simulink model "Plant"  (R2025a)
settings: Solver=ode4  StartTime=0.0  StopTime=10  FixedStep=2e-4  RelTol=1e-3
model workspace (MAT data in the model file):
  phTyreNomPres = 262000
  plantVx0 = 68.8718280662
undefined symbols (not defined in the file): pt, sus, tyreParamVec, vp
libraries: AeroActuators x2, vehdynlibeom x1
(part 1 of 2)
Description:
  | ARFWr RT plant (T2.2 skeleton). 1 kHz, ode4, model-reference target for ARFWr_Sim.
  | 
  | FRAME CONVENTION -- READ FIRST.
  | The rigid body is the VDB "Vehicle Body 6DOF" block, which wraps the Aerospace
  | 6DOF (Euler Angles) block and therefore uses SAE J670 body axes: x FORWARD,
  | y RIGHT, z DOWN. This was MEASURED on the live R2025a block during T2.2, not
  | assumed: FSusp(3,:) = -[Ff Ff Fr Fr] holds the body in exact static equilibrium
  | (all six DOF stay at zero), while +z of the same magnitude doubles the
  | gravitational fall. FSusp/MSusp are 3-by-4, columns ordered [FL FR RL RR]
  | (measured: an extra UP force on column 1 rolls the body left-side-up).
  | 
  | Everything else in this repo -- Scripts/vehModel.m, the ARFWr reactive law,
  | simulink/ecu/tvAllocStep.m, the curv2cart racing line -- is ISO 8855:
  | x FORWARD, y LEFT, z UP, yaw rate r > 0 = LEFT turn.
  | 
  | This model therefore works INTERNALLY in the SAE frame and MIRRORS at the bus
  | boundary (Vehicle State Bus subsystem):  y, vy, ay, psi, r, z, roll all negate;
  | pitch does not (the mirror is about the x-z plane). Corner LABELS fl/fr/rl/rr
  | are physical and never flip.
  | 
  | PLACEHOLDERS in this model (see the model workspace, all prefixed ph*):
  |   phTyreNomPres        tyre block nominal pressure (inert: driven AT NOMPRES)
  | T3.2 replaced the tyre placeholder with the Zenvo MF5.2 law; T3.4 replaced the aero placeholder with the live ride-height map, so the constant-coefficient phAeroClF/phAeroClR and the phIxx/phIyy inertia placeholders are deleted -- the inertia tensor is now the supplier one (inrt.Iveh).
settings Model: DataDictionary=ARFWr_RT.sldd  Creator=ASUS  LastModifiedBy=ASUS
settings DataIOCC: SignalLoggingName=plantLog
settings DebuggingCC: AlgebraicLoopMsg=error  UnconnectedInputMsg=error  UnconnectedOutputMsg=error  UnconnectedLineMsg=error

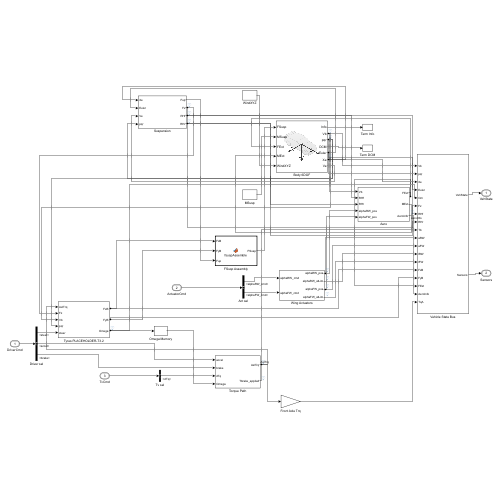
[thumbnail: Simulink's stored preview of the top-level diagram]
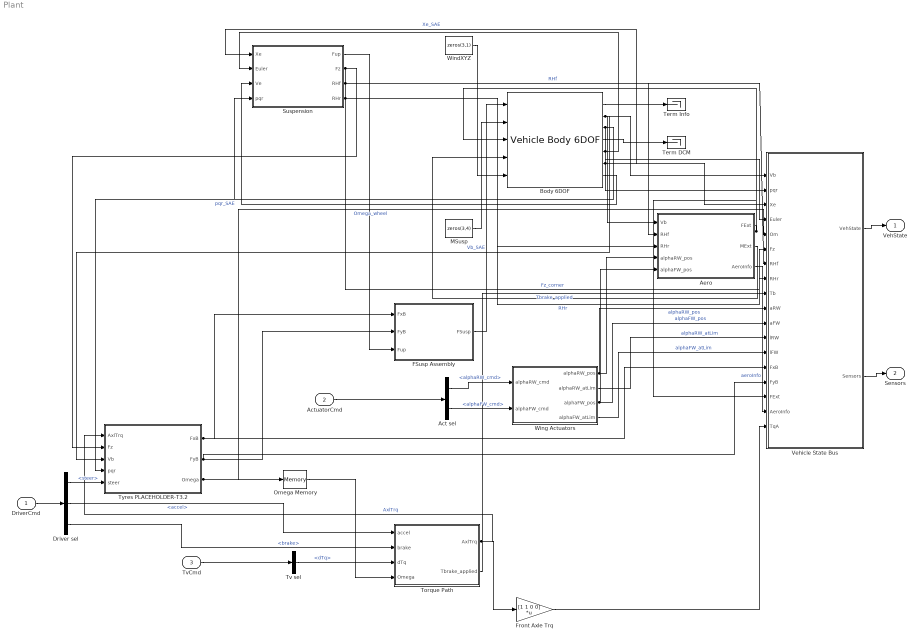
== system Plant ==
  DriverCmd : Inport  Description=Driver / scenario demand. ISO 8855 steer (+ = LEFT road-wheel angle, rad), accel and brake in 0..1.  OutDataTypeStr=Bus: DriverCmdBus
  ActuatorCmd : Inport  Description=Wing angle demands out of AeroECU. The two wing ACTUATORS live here in the plant (design decision 7: they are the HIL seam, replaced by hardware later), so the ECU commands and the plant reports positions.  Port=2  OutDataTypeStr=Bus: ActuatorCmdBus
  TvCmd : Inport  Description=Torque-vectoring differential torque (TvCmdBus.dTq), driven by the AeroECU allocator in the closed-loop harness. The Torque Path applies it as a front-axle left/right split: AxlTrq_FR - AxlTrq_FL = dTq.  Port=3  OutDataTypeStr=Bus: TvCmdBus
  Act sel : BusSelector  OutputSignals=alphaRW_cmd,alphaFW_cmd
  Aero : Subsystem  Description=|
      | LIVE ride-height aerodynamics (T3.4). Replaced the T2.2 constant-coefficient placeholder; the four signals that used to be terminated here (RHf, RHr, alphaRW_pos, alphaFW_pos) are now CONSUMED, so the wings finally do something.
      | 
      | WHAT IT COMPUTES, per step (formulas and derivation: simulink/aero/aeroLiveEval.m):
      |   ClF = interp2(base map)(RHf,RHr) + blend_RW(alphaRW).dClF + blend_FW(alphaFW).dClFadd
      |   ClR = interp2(base map)(RHf,RHr) + blend_RW(alphaRW).dClR + blend_FW(alphaFW).dClRadd
      |   Cd  = vp.Cd0 + (dCdA_RW(alphaRW) + dCdA_FW(alphaFW))/vp.A
      | The base map is the MID (0 deg both wings) ride-height grid, indexed at the INSTANTANEOUS ride height the Suspension subsystem publishes -- not at a quasi-statically collapsed one. That is the whole reason a 6-DOF plant is worth building: the offline solver bakes ride height out of the model (one aeroCollapse fixed point per wing node, fitted to a speed-only curve), and cannot see a transient attitude.
      | 
      | FORCE APPLICATION (SAE body axes here: x fwd, y RIGHT, z DOWN).
      | FExt acts at the CG (measured on the VDB block in T2.2: an FExt(1) step produces exactly zero pitch), so both the front/rear lift split AND the drag height split have to be re-expressed as explicit MExt pitch moments:
      |   lift  DFf at x = +vp.l_f, DFr at x = -vp.l_r   ->  M_y = -l_f*DFf + l_r*DFr
      |   drag  body part vp.Cd0 at vp.hcg  ->  no moment (it acts at the CG height)
      |         wing increment (Cd - Cd0) at vp.hw  ->  M_y = +(vp.hw - vp.hcg)*Fdrag_rw
      | This is the vp.hw term build_plant.m's placeholder description said T3.4 would add, and it is the same f_drag0/f_dragRW height split Scripts/vehModel.m:603-604 defines.
      | 
      | KNOWN LIMITATION, read before believing a deployed-front-wing number. The offline model builds the FRONT-wing layer with liftMode = 'additive' (Functions/rwAeroMap2D.m), i.e. the FW lift deltas are added to a ride-height trajectory collapsed with the FW delta set to ZERO -- deliberately, because the FW-deployed CFD states fall outside aeroCollapse's convergence envelope. A live plant cannot open that loop: here the FW lift delta really does extend the front suspension, which raises the nose, which the base map answers with LESS front downforce. See docs / the T3.4 report for the measured size of that divergence.
  Body 6DOF : vehdynlibeom/Vehicle Body 6DOF  Description=|  extPos=on  extVel=on  extEuler=on  extRotRate=on  htchFMode=off  htchMMode=off  m=vp.m  a=vp.l_f  b=vp.l_r  d=0  h=vp.hcg  dh=1  hl=0  hh=0.1  Xe_o=[0,0,0]  xbdot_o=[plantVx0,0,0]  eul_o=[0,0,0]  p_o=[0,0,0]  Iveh=inrt.Iveh  w=[vp.t, vp.t]  z1m=0  z1R=[-.25,.125,.15]  z1I=[1.4,-.2,.1;-.2,1.4,.1;.1,.1,2.25].*0  z2m=0  z2R=[1.4,0,.8]  z2I=[1.4,-.2,.1;-.2,1.4,.1;.1,.1,2.25].*0  z3m=0  z3R=[.75,-.5,.4]  z3I=[5,-.1,-2;-2,9,.1;-.1,.1,6].*0  z4m=0  z4R=[.75,.5,.4]  z4I=[5,-.1,-2;-2,9,.1;-.1,.1,6].*0  z5m=0  z5R=[1.25,-.5,.4]  z5I=[5,-.1,-2;-2,9,.1;-.1,.1,6].*0  z6m=0  z6R=[1.25,-.5,.4]  z6I=[5,-.1,-2;-2,9,.1;-.1,.1,6].*0  z7m=0  z7R=[2,0,.25]  z7I=[1.4,-.2,.1;-.2,1.4,.1;.1,.1,2.25].*0  Af=vp.A  Cd=0  Cl=0  Cpm=0  beta_w=[0:0.001:0.01]  Cs=[0:0.01:0.1]  Cym=[0:0.001:0.01]  Pabs=101325  extTamb=off  Tair=273  g=vp.g  xdot_tol=.1  longOff=0  latOff=0  vertOff=0  wrapAng=on  aMode=2
      | VDB Vehicle Body 6DOF -- SAE J670 body axes (x fwd, y RIGHT, z DOWN), measured in T2.2. See the model description for the full convention note.
      | 
      | h = vp.hcg (not vp.hcg - vp.Rw) ON PURPOSE. The mask calls h the "vertical distance from centre of mass to axle plane", i.e. the height at which FSusp columns are applied. This model has no unsprung mass and no suspension block, so what is fed through FSusp rows 1-2 is the TYRE CONTACT-PATCH force, whose true application height is ground level = vp.hcg below the CG. Setting h = vp.hcg therefore gives the correct roll/pitch moment arm (verified: a pure -x force at the corners produces nose-down pitch; a +y force rolls the body left-side-down, i.e. outboard).
      | 
      | The block's OWN aero model is switched off (Cd = Cl = Cpm = 0) so the Aero subsystem is the single owner of aerodynamic force -- otherwise T3.4 would have to fight a second, single-point aero model that cannot split lift per axle. Af is still set to vp.A so a reader sees the right reference area.
      | 
      | Iveh = inrt.Iveh (T3.4), the SUPPLIER tensor diag([500 2500 2900]) kg.m^2 from Zenvo's vehicle-parameter workbook, sheet "Vehicle", "Vehicle Inertia" rows 32-34. The T2.2 phIxx/phIyy placeholders are gone: they were built on the premise that no supplier Ixx/Iyy existed, and it does -- see simulink/params/inertiaBorrowed.m, which also carries the radius-of-gyration cross-check (a calibrated solid box predicts the two to within +1.5 % and +4.0 %). vp.I_z (2900) is the Izz entry of that same row block, so all three now come from one source.
  Driver sel : BusSelector  OutputSignals=steer,accel,brake
  FSusp Assembly : MATLAB Function  Description=Builds the VDB Vehicle Body 6DOF FSusp input: a 3-by-4 matrix, rows = force along vehicle-fixed [x; y; z], columns = [FL FR RL RR] (both MEASURED on the live block, see the model description). Rows 1-2 are the tyre contact-patch forces in body axes; row 3 is -Fup, because the suspension pushes the body UP and +z is DOWN.  TreatAsAtomicUnit=on
  Front Axle Trq : Gain  Description=|  Gain=[1 1 0 0]  Multiplication=Matrix(K*u)
      | TqAxle for the TV allocator: the NOMINAL (pre-TV) total FRONT-axle wheel torque,
      | AxlTrq(FL) + AxlTrq(FR), in Nm, drive plus brake, signed.
      | 
      | WHY THE SUM IS THE PRE-TV QUANTITY, exactly and not approximately: Torque Path's
      | torqueStep forms AxlTrq(1) = TwF/2 - dTq/2 + Tbf and AxlTrq(2) = TwF/2 + dTq/2 + Tbf,
      | so the +/-dTq/2 shift CANCELS in the sum by construction and this signal equals
      | TwF + 2*Tbf for any dTq. That is precisely what simulink/ecu/tvAllocStep.m's headroom
      | clamp expects -- headroom = 2*(perSideCapNm - |TqAxle|/2) is the room each side has
      | left ABOVE its symmetric TqAxle/2 baseline -- so feeding the post-TV per-wheel torque
      | instead would double-count the shift the clamp is sizing.
      | 
      | It carries the BRAKE share too (Tbf), not just the drive share, because the per-wheel
      | motor torque a TV shift has to fit alongside is the whole signed wheel torque.
      | 
      | ALGEBRAIC LOOP: this closes dTq -> Torque Path -> here -> SensorBus -> ECU -> dTq. It
      | is broken OUTSIDE the Plant, by the one-sample Memory in ARFWr_Sim/ECU Sensor Latency
      | (the same block that already breaks the vx/r path), not by anything here.
  MSusp : Constant  Description=Suspension MOMENTS about each hard point. Zero: this skeleton applies pure forces at the contact patches, and the resulting body moments come from the hard-point lever arms the block already applies.  Value=zeros(3,4)
  Omega Memory : Memory  Description=|
      | ALGEBRAIC-LOOP BREAK. The VDB Combined Slip Wheel 2DOF block's Omega output has direct feedthrough from its AxlTrq input (through the block's own Wheel Module clutch), so feeding Omega back into the Torque Path's power cap closes an algebraic loop that Simulink refuses to solve (the clutch updates state while computing outputs).
      | 
      | Breaking it with a one-major-step Memory is both the standard fix and the physically honest one: the power cap min(Tmax*gear, Pmax/mean(Om)) is an inverter/ECU calculation that in hardware necessarily uses the PREVIOUS speed sample. At 1 ms the lag is negligible against wheel-speed dynamics, and the formula itself is unchanged from Scripts/vehModel.m:655 + Parameters/Powertrain.m:12. Initial condition 0 rad/s is the standstill state, where the cap is the torque branch (Tmax*gear) anyway -- the Om floor in torqueStep guards the division.
  Suspension : Subsystem  Description=|
      | Four independent corners: linear wheel-rate spring (vp.kwf/vp.kwr), borrowed damper (sus.cDamp_f/sus.cDamp_r) and borrowed anti-roll bar (sus.kArb_f/sus.kArb_r) -- see simulink/params/suspensionBorrowed.m for the OptimumG derivation and provenance tags.
      | 
      | MODELLING LIMITATION (skeleton): rigid tyres, no unsprung mass, no tyre vertical stiffness, flat ground, and no roll-centre/jacking geometry. Corner compression is purely the body attitude change at that corner, so load transfer here is the through-the-springs component only. The geometric (roll-centre) component is missing; vp.hRCf/vp.hRCr exist and a later task can add it. Also: the model starts in exact static equilibrium (the static corner load is carried explicitly), so compression = 0 IS the reference attitude and RHf/RHr start at vp.RHf0/vp.RHr0.
      | 
      | RIDE HEIGHT UNITS: vp.RHf0 = 85 and vp.RHr0 = 95 are MILLIMETRES (Parameters/vehParams.m; Functions/aeroCollapse.m:23-25 documents the map grid as mm). Compression is metres, hence the x1000. CLOSED IN T3.4: the Params constant now carries vp.RHfU/vp.RHrU (the v = 0 unloaded heights) instead of vp.RHf0/vp.RHr0 (the v = 10 m/s nominal heights), so zero compression means the same physical attitude here as in Functions/aeroCollapse.m.
  Term DCM : Terminator
  Term Info : Terminator
  Torque Path : Subsystem  Description=|
      | Simplified torque path, mirroring Scripts/vehModel.m:660-663 (the pt.ATD == 0 ladder) plus the front-axle TV shift of simulink/ecu/tvAllocStep.m.
      | SOURCES OF THE TWO SPLIT CONSTANTS (found by grep for T2.2 -- pt.ATD is NOT set by Parameters/Powertrain.m, it is set by Scripts/userOpts.m, so the plant reproduces the fixed AWD split, not an ATD ladder):
      |   vp.Tdist = 0.78  Parameters/vehParams.m:20 -- REAR torque fraction. Sized in Parameters/Powertrain.m:71-75 so the fixed split never demands more than the front axle's 300 kW (2 x 150 kW e-motors) out of the 1068 kW rear path.
      |   vp.brkB  = 0.65  Parameters/vehParams.m:19 -- FRONT brake-force fraction, Zenvo sheet "mechanical pressure bias front 0.65 nominally".
      | Both are read by NAME from the base workspace via the Params constant.
  Tv sel : BusSelector  OutputSignals=dTq
  Tyres PLACEHOLDER-T3.2 : Subsystem  Description=|
      | TYRES -- real Zenvo MF5.2, applied T3.2. (The block name still carries the PLACEHOLDER-T3.2 tag only because renaming a subsystem breaks every stored signal-logging path and every task brief that references it.)
      | 
      | The four VDB "Combined Slip Wheel 2DOF" blocks are GONE, replaced by tyreStep, a direct implementation of Functions/tyreMFnum.m, plus an explicit wheel-spin integrator. See tyreStep's own description for the measured gate-1 evidence that forced this, and TyreParams for how the confidential coefficients reach the model without being stored in it.
      | 
      | --- superseded notes from the placeholder era, kept for provenance ---
      | *** PLACEHOLDER-T3.2 *** The two VDB "Combined Slip Wheel 2DOF" blocks inside carry their BUILT-IN DEFAULT Magic Formula 6.2 coefficient set (the block's "Mid-size passenger car 235/45R18"), NOT the Zenvo MF5.2 data. Peak mu is therefore about 0.81 and the car is far less grippy than the real vehicle. T3.2 replaces exactly this: mf52ToVDB(vp.tyre_f) / mf52ToVDB(vp.tyre_r) set_param'd onto the two blocks -- one block per axle is deliberate, because that is the granularity of the supplier data (vp.tyre_f / vp.tyre_r). THE SWAP IS ONE SUBSYSTEM: nothing outside this boundary changes.
      | 
      | CONFIDENTIALITY: no tyre coefficient value is stored in this .slx. T3.2 must apply them by set_param from vp.tyre_f/vp.tyre_r at load time, or the .slx would carry supplier data in its dialogs (project confidentiality rule).
      | 
      | STRUCTURAL settings applied here (vehicle geometry / wiring choices, NOT tyre data, and identical to what simulink/validation/validateTyreBlocks.m sets for gate 1): vertType = None (normal load comes in through Fext, so the suspension owns the vertical chain), BrakeType = None (brake torque is carried signed inside AxlTrq, matching vehModel.m's T_fl..T_rr), turnslip = off, and a rigid effective rolling radius equal to vp.Rw (UNLOADED_RADIUS = vp.Rw, Q_RE0 = 1, BREFF = DREFF = FREFF = 0). IYY is set to vp.Jw so wheel spin-up matches the MLTP model. plySteer is also OFF: the default tyre's ply-steer/conicity shift terms (PHY1, PVY1, ...) are identical on both sides of the car, so they push a nominally symmetric straight-line run sideways -- measured in T2.2, the untouched default reached |vy| = 11.8 m/s and |r| = 3.2 rad/s on a zero-steer full-throttle run. mf52ToVDB.m sets every shift term to exactly zero anyway, so turning ply steer off makes the placeholder STRUCTURALLY match what T3.2 installs.
      | 
      | LIBRARY PATH NOTE for T3.2: the loadable path is 'vehdynlibtire/Combined Slip Wheel 2DOF'. The path currently hardcoded in validateTyreBlocks.m:299, 'vdynblks/Wheels and Tires/Combined Slip Wheel 2DOF', does NOT load in R2025a (there is no loadable block diagram named vdynblks) -- that is its own VERIFY #1 and must be fixed before gate 1 runs.
      | 
      | T3.2 WIRING FIX (2026-09-02) -- MEASURED ROOT CAUSE.
      | Setting BrakeType = 'None' does TWO things to this block's input port list: it
      | removes BrkPrs (10 ports -> 9) AND it SWAPS the relative order of Gnd and Fext.
      | Measured on the live R2025a block:
      |   defaults           (10): BrkPrs AxlTrq Vx Vy Camber YawRate Prs Gnd Fext ScaleFctrs
      |   BrakeType = None    (9): AxlTrq Vx Vy Camber YawRate Prs Fext Gnd ScaleFctrs
      | build_plant.m accounted for the dropped BrkPrs but not the swap, so it wired the
      | Gnd constant (0) into port 7 = Fext and the suspension normal load DFzc into
      | port 8 = Gnd. With vertType = None the Gnd input is inert, so every tyre ran at
      | Fz = 0 (T2.3 measured tyre Fz output exactly 0.0 while VehStateBus.Fz_rl read
      | 4479-5085 N), produced ~30-100 N instead of thousands, and the wheels spun up
      | until the My Relaxation integrator went non-finite (t = 0.1825 s at 25%% throttle
      | from rest -- re-measured on the committed file by T3.2).
      | Ports 7/8 are now DFzc -> Fext, Gnd constant -> Gnd, and each block's own Fz
      | output is NAMED and LOGGED (Fz_tyre_FL..RR) so this class of fault is visible.
      | NEVER wire this block by port NUMBER against the documented order: resolve the
      | index from the live port names (find_system for its internal Inport blocks).
  Vehicle State Bus : Subsystem  Description=|
      | Assembles VehStateBus and SensorBus, and applies the SAE -> ISO 8855 mirror documented in the model description. This subsystem is the ONLY place the sign flip happens; nothing downstream (AeroECU, DriverPath, the reactive law, the TV allocator) ever sees SAE-framed signals.
      | 
      | SensorBus contract, checked against Functions/rwVelocityTarget.m's brakeSwitch: Tbrake is passed SIGNED (<= 0 while braking) -- brakeSwitch applies tbSign = -1 itself and deliberately avoids abs() -- and TbMax is the POSITIVE magnitude cap vp.Tbrake_max = 7000 Nm. TbMax > 0 ALWAYS: the law's onset width is w1frac*TbMax, so a negative or zero TbMax would invert or divide-by-zero the brake trigger.
  WindXYZ : Constant  Description=Wind velocity [m/s]. Zero: still air.  Value=zeros(3,1)
  Wing Actuators : Subsystem  Description=Both wing actuators: first-order lag (act.tau) -> rate limit (act.rateLim, +-25 deg/s Zenvo directive) -> travel clamp. Library instances of AeroActuators/ActuatorWing (T1.4). Positions are LOGGED and published on VehStateBus; T2.2 does NOT feed them to the aero -- the Aero subsystem receives them and terminates them, which is the seam T3.4 opens.
  VehState : Outport  Description=Full plant state, ISO 8855. See the sldd bus description.  OutDataTypeStr=Bus: VehStateBus
  Sensors : Outport  Description=The four signals AeroECU consumes, ISO 8855, Tbrake SIGNED.  Port=2  OutDataTypeStr=Bus: SensorBus
  wires:
  Omega Memory/1 -> Torque Path/4(Omega)
  DriverCmd/1 -> Driver sel/1
  TvCmd/1 -> Tv sel/1
  Driver sel/1 -> Tyres PLACEHOLDER-T3.2/5(steer)  "<steer>"
  Driver sel/2 -> Torque Path/1(accel)  "<accel>"
  Suspension/4(RHr) -> Aero/3(RHr), Vehicle State Bus/8(RHr)  "RHr"
  Tyres PLACEHOLDER-T3.2/2(FyB) -> FSusp Assembly/2(FyB), Vehicle State Bus/15(FyB)
  Wing Actuators/1(alphaRW_pos) -> Vehicle State Bus/10(aRW), Aero/4(alphaRW_pos)  "alphaRW_pos"
  Body 6DOF/7 -> Suspension/3(Ve)
  Tyres PLACEHOLDER-T3.2/1(FxB) -> Vehicle State Bus/14(FxB), FSusp Assembly/1(FxB)
  Body 6DOF/3 -> Suspension/4(pqr), Vehicle State Bus/2(pqr), Tyres PLACEHOLDER-T3.2/4(pqr)  "pqr_SAE"
  Driver sel/3 -> Torque Path/2(brake)  "<brake>"
  Tyres PLACEHOLDER-T3.2/3(Omega) -> Vehicle State Bus/5(Om), Omega Memory/1  "Omega_wheel"
  Suspension/1(Fup) -> FSusp Assembly/3(Fup)
  Suspension/2(Fz) -> Tyres PLACEHOLDER-T3.2/2(Fz), Vehicle State Bus/6(Fz)  "Fz_corner"
  Suspension/3(RHf) -> Aero/2(RHf), Vehicle State Bus/7(RHf)  "RHf"
  ActuatorCmd/1 -> Act sel/1
  Torque Path/1(AxlTrq) -> Tyres PLACEHOLDER-T3.2/1(AxlTrq), Front Axle Trq/1  "AxlTrq"
  Tv sel/1 -> Torque Path/3(dTq)  "<dTq>"
  WindXYZ/1 -> Body 6DOF/5
  MSusp/1 -> Body 6DOF/2
  FSusp Assembly/1(FSusp) -> Body 6DOF/1
  Vehicle State Bus/1(VehState) -> VehState/1
  Act sel/1 -> Wing Actuators/1(alphaRW_cmd)  "<alphaRW_cmd>"
  Act sel/2 -> Wing Actuators/2(alphaFW_cmd)  "<alphaFW_cmd>"
  Torque Path/2(Tbrake_applied) -> Vehicle State Bus/9(Tb)  "Tbrake_applied"
  Aero/2(MExt) -> Body 6DOF/4
  Body 6DOF/1 -> Term Info/1
  Body 6DOF/2 -> Tyres PLACEHOLDER-T3.2/3(Vb), Aero/1(Vb), Vehicle State Bus/1(Vb)  "Vb_SAE"
  Body 6DOF/4 -> Term DCM/1
  Body 6DOF/5 -> Suspension/2(Euler), Vehicle State Bus/4(Euler)
  Body 6DOF/6 -> Suspension/1(Xe), Vehicle State Bus/3(Xe)  "Xe_SAE"
  Wing Actuators/2(alphaRW_atLim) -> Vehicle State Bus/12(lRW)  "alphaRW_atLim"
  Wing Actuators/3(alphaFW_pos) -> Vehicle State Bus/11(aFW), Aero/5(alphaFW_pos)  "alphaFW_pos"
  Wing Actuators/4(alphaFW_atLim) -> Vehicle State Bus/13(lFW)  "alphaFW_atLim"
  Aero/1(FExt) -> Body 6DOF/3, Vehicle State Bus/16(FExt)
  Vehicle State Bus/2(Sensors) -> Sensors/1
  Aero/3(AeroInfo) -> Vehicle State Bus/17(AeroInfo)  "aeroInfo"
  Front Axle Trq/1 -> Vehicle State Bus/18(TqA)

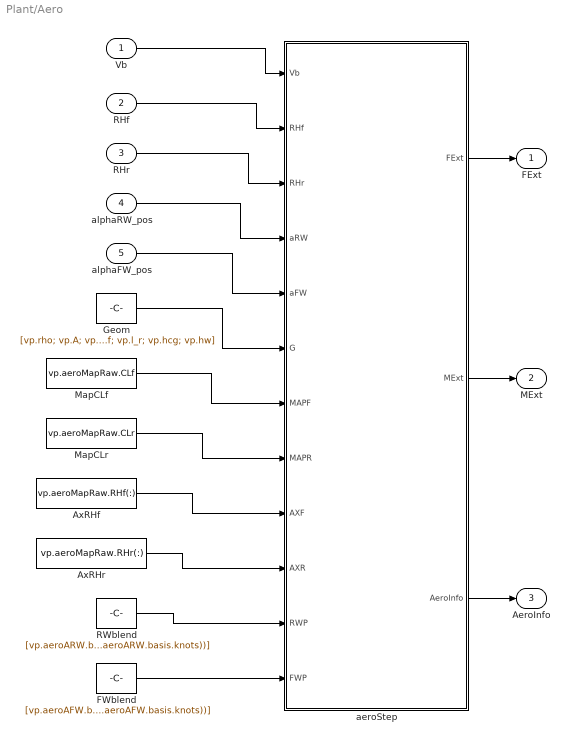
== system Plant/Aero ==
  Vb : Inport
  RHf : Inport  Port=2
  RHr : Inport  Port=3
  alphaRW_pos : Inport  Port=4
  alphaFW_pos : Inport  Port=5
  AxRHf : Constant  Description=Front ride-height axis of the raw map [mm], ascending. Grid edges are where aeroStep clamps.  Value=vp.aeroMapRaw.RHf(:)
  AxRHr : Constant  Description=Rear ride-height axis of the raw map [mm], ascending.  Value=vp.aeroMapRaw.RHr(:)
  FWblend : Constant  Description=|  Value=[vp.aeroAFW.basis.knots(:).'; repmat(vp.aeroAFW.basis.wb,1,numel(vp.aeroAFW.basis.knots)); vp.aeroAFW.dClFadd(:).'; vp.aeroAFW.dClRadd(:).'; vp.aeroAFW.dCdA(:).'; reshape(permute(vp.aeroAFW.basis.C,[2 1 3]),[],numel(vp.aeroAFW.basis.knots))]
      | Cardinal-basis blend parameters for the FRONT wing, packed as a matrix with one COLUMN per map node. Row layout, read by index inside aeroStep:
      |   row 1        alphaNodes  [deg]        (the node angles, ascending)
      |   row 2        basis.wb    [deg]        (tanh switch width, replicated across columns)
      |   row 3        dClFadd     [-]          (front-axle lift delta at that node)
      |   row 4        dClRadd     [-]          (rear-axle  lift delta at that node)
      |   row 5        dCdA        [m^2]        (drag-area delta at that node)
      |   rows 6..end  basis.C, permuted to [4*(n-1) x n]: rows (j-1)*4+1..(j-1)*4+4 are the four
      |                Horner coefficients (highest order first) of polynomial segment j at node i.
      | 
      | The blend itself is Functions/rwBasisWeights.m's tanh switch stack -- pure tanh/multiply/add/Horner arithmetic, which is why it ports to a codegen MATLAB Function block unchanged. n and the segment count are read from the SIGNAL DIMENSIONS, so this stays correct if the map ever changes node count.
      | 
      | .dClFadd/.dClRadd (NOT .dClF/.dClR) is correct for the FW layer: it is built with liftMode = 'additive' (Parameters/vehParams.m, rwMandate 5/6/7), where the *add fields ARE the per-node constant shift by construction and .dClF/.dClR are zeros. Same choice Functions/rwAeroMapEvalNum.m makes in its own FW-layer accumulation.
  Geom : Constant  Description=|  Value=[vp.rho; vp.A; vp.Cd0; vp.l_f; vp.l_r; vp.hcg; vp.hw]
      | Scalar aero geometry, IN THIS ORDER (aeroStep reads them by index):
      | 1 vp.rho  air density [kg/m^3]
      | 2 vp.A    fixed reference frontal area [m^2] -- every Cl/Cd in this model is on it
      | 3 vp.Cd0  body drag coefficient [-], the wing-angle-independent part
      | 4 vp.l_f  CG -> front axle [m]   (lift application point, front)
      | 5 vp.l_r  CG -> rear  axle [m]   (lift application point, rear)
      | 6 vp.hcg  CG height [m]          (body-drag application height)
      | 7 vp.hw   rear-wing height [m]   (wing-drag-increment application height)
  MapCLf : Constant  Description=Raw ride-height FRONT lift map, [numel(RHf) x numel(RHr)] (rows = front ride height, columns = rear ride height), MID wing state (alphaRW = alphaFW = 0). This is the same grid Functions/aeroCollapse.m interpolates inside its quasi-static fixed point -- Parameters/aeroMap_Tur.mat, loaded ONCE at project startup by simulink/params/loadVehicleParams.m and reachable here as vp.aeroMapRaw. The block never calls load().  Value=vp.aeroMapRaw.CLf
  MapCLr : Constant  Description=Raw ride-height REAR lift map, same shape and provenance as MapCLf.  Value=vp.aeroMapRaw.CLr
  RWblend : Constant  Description=|  Value=[vp.aeroARW.basis.knots(:).'; repmat(vp.aeroARW.basis.wb,1,numel(vp.aeroARW.basis.knots)); vp.aeroARW.dClF(:).'; vp.aeroARW.dClR(:).'; vp.aeroARW.dCdA(:).'; reshape(permute(vp.aeroARW.basis.C,[2 1 3]),[],numel(vp.aeroARW.basis.knots))]
      | Cardinal-basis blend parameters for the REAR wing, packed as a matrix with one COLUMN per map node. Row layout, read by index inside aeroStep:
      |   row 1        alphaNodes  [deg]        (the node angles, ascending)
      |   row 2        basis.wb    [deg]        (tanh switch width, replicated across columns)
      |   row 3        dClF        [-]          (front-axle lift delta at that node)
      |   row 4        dClR        [-]          (rear-axle  lift delta at that node)
      |   row 5        dCdA        [m^2]        (drag-area delta at that node)
      |   rows 6..end  basis.C, permuted to [4*(n-1) x n]: rows (j-1)*4+1..(j-1)*4+4 are the four
      |                Horner coefficients (highest order first) of polynomial segment j at node i.
      | 
      | The blend itself is Functions/rwBasisWeights.m's tanh switch stack -- pure tanh/multiply/add/Horner arithmetic, which is why it ports to a codegen MATLAB Function block unchanged. n and the segment count are read from the SIGNAL DIMENSIONS, so this stays correct if the map ever changes node count.
      | 
      | .dClF/.dClR (not .dClFadd/.dClRadd) is correct for the RW map: it is built with liftMode = 'collapse', where .dClF/.dClR are the values actually handed to Functions/aeroCollapse.m -- i.e. exactly the constant its clfFun/clrFun add to this same base grid -- and the *add fields are zeros.
  aeroStep : MATLAB Function  Description=Live ride-height aero (T3.4). Codegen-safe port of simulink/aero/aeroLiveEval.m's formulas -- see that file's header for the derivation and for why the RT plant interpolates the RAW ride-height grid instead of the offline solver's pre-collapsed, speed-only fits. The reference implementation itself is NOT codegen-safe (persistent + load + cell arrays); this is a re-implementation of the same arithmetic, gate-checked against it by simulink/validation/validateAeroLive.m section (C).  TreatAsAtomicUnit=on
  FExt : Outport
  MExt : Outport  Port=2
  AeroInfo : Outport  Description=Aero diagnostics, 4x1 = [ClF; ClR; Cd; clampCode]. Published on VehStateBus as aeroClF/aeroClR/aeroCd/aeroClamp. clampCode is a bit field: +1 RHf clamped to the map grid, +2 RHr clamped, +4 alphaRW clamped to the node range, +8 alphaFW clamped.  Port=3
  wires:
  aeroStep/3(AeroInfo) -> AeroInfo/1
  Vb/1 -> aeroStep/1(Vb)
  RHf/1 -> aeroStep/2(RHf)
  RHr/1 -> aeroStep/3(RHr)
  alphaRW_pos/1 -> aeroStep/4(aRW)
  alphaFW_pos/1 -> aeroStep/5(aFW)
  Geom/1 -> aeroStep/6(G)
  MapCLr/1 -> aeroStep/8(MAPR)
  MapCLf/1 -> aeroStep/7(MAPF)
  AxRHf/1 -> aeroStep/9(AXF)
  AxRHr/1 -> aeroStep/10(AXR)
  RWblend/1 -> aeroStep/11(RWP)
  FWblend/1 -> aeroStep/12(FWP)
  aeroStep/1(FExt) -> FExt/1
  aeroStep/2(MExt) -> MExt/1

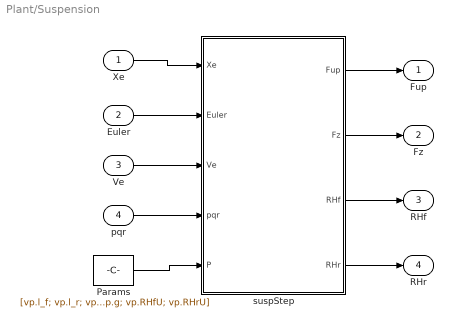
== system Plant/Suspension ==
  Xe : Inport
  Euler : Inport  Port=2
  Ve : Inport  Port=3
  pqr : Inport  Port=4
  Params : Constant  Description=|  Value=[vp.l_f; vp.l_r; vp.t; vp.hcg; vp.kwf; vp.kwr; sus.cDamp_f; sus.cDamp_r; sus.kArb_f; sus.kArb_r; vp.m; vp.g; vp.RHfU; vp.RHrU]
      | Suspension parameters, IN THIS ORDER (suspStep reads them by index):
      |  1 vp.l_f        CG->front axle [m]                Parameters/vehParams.m:55
      |  2 vp.l_r        CG->rear  axle [m]                Parameters/vehParams.m:56
      |  3 vp.t          track width [m]                   Parameters/vehParams.m:49
      |  4 vp.hcg        CG height [m]                     Parameters/vehParams.m:58
      |  5 vp.kwf        front wheel rate [N/m]            Parameters/vehParams.m:72
      |  6 vp.kwr        rear  wheel rate [N/m]            Parameters/vehParams.m:73
      |  7 sus.cDamp_f   front damper [N.s/m]   BORROWED    simulink/params/suspensionBorrowed.m
      |  8 sus.cDamp_r   rear  damper [N.s/m]   BORROWED
      |  9 sus.kArb_f    front ARB [Nm/rad]     BORROWED
      | 10 sus.kArb_r    rear  ARB [Nm/rad]     BORROWED
      | 11 vp.m          total mass [kg]                   Parameters/vehParams.m:45
      | 12 vp.g          gravity [m/s^2]                   Parameters/vehParams.m:35
      | 13 vp.RHfU       front ride height at v = 0 [mm]   simulink/params/loadVehicleParams.m
      | 14 vp.RHrU       rear  ride height at v = 0 [mm]
      |    T3.4 closed the offset build_plant.m flagged: vp.RHf0/vp.RHr0 (85/95 mm) are the
      |    nominal heights AT v = 10 m/s (Functions/aeroCollapse.m anchors its fixed point
      |    there), but zero spring compression in this model is the STATIC, no-aero state.
      |    vp.RHfU/vp.RHrU are aeroCollapse's own unloaded heights (85.429 / 95.278 mm),
      |    read back from the alpha = 0 node, so the plant and the offline map agree at
      |    10 m/s instead of being 0.43 / 0.28 mm apart.
  suspStep : MATLAB Function  TreatAsAtomicUnit=on
  Fup : Outport
  Fz : Outport  Port=2
  RHf : Outport  Port=3
  RHr : Outport  Port=4
  wires:
  Params/1 -> suspStep/5(P)
  Ve/1 -> suspStep/3(Ve)
  Xe/1 -> suspStep/1(Xe)
  suspStep/2(Fz) -> Fz/1
  Euler/1 -> suspStep/2(Euler)
  pqr/1 -> suspStep/4(pqr)
  suspStep/1(Fup) -> Fup/1
  suspStep/3(RHf) -> RHf/1
  suspStep/4(RHr) -> RHr/1

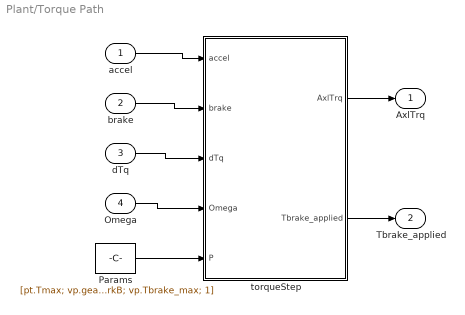
== system Plant/Torque Path ==
  accel : Inport
  brake : Inport  Port=2
  dTq : Inport  Port=3
  Omega : Inport  Port=4
  Params : Constant  Description=|  Value=[pt.Tmax; vp.gear; pt.Pmax; vp.Tdist; vp.brkB; vp.Tbrake_max; 1]
      | Torque-path parameters, IN THIS ORDER (torqueStep reads them by index):
      | 1 pt.Tmax        machine-side torque cap [Nm]      Parameters/Powertrain.m:80
      | 2 vp.gear        effective single ratio [-]        Parameters/Powertrain.m:67
      | 3 pt.Pmax        wheel-side power cap [W]          Parameters/Powertrain.m:53
      | 4 vp.Tdist       REAR torque fraction [-]          Parameters/vehParams.m:20
      | 5 vp.brkB        FRONT brake fraction [-]          Parameters/vehParams.m:19
      | 6 vp.Tbrake_max  brake channel magnitude cap [Nm]  Parameters/vehParams.m:344
      | 7 Om floor       [rad/s] guards Pmax/Om at standstill -- a numerical guard, not
      |                  vehicle data, so it is the one literal in this vector.
  torqueStep : MATLAB Function  TreatAsAtomicUnit=on
  AxlTrq : Outport
  Tbrake_applied : Outport  Port=2
  wires:
  torqueStep/1(AxlTrq) -> AxlTrq/1
  accel/1 -> torqueStep/1(accel)
  brake/1 -> torqueStep/2(brake)
  torqueStep/2(Tbrake_applied) -> Tbrake_applied/1
  dTq/1 -> torqueStep/3(dTq)
  Omega/1 -> torqueStep/4(Omega)
  Params/1 -> torqueStep/5(P)

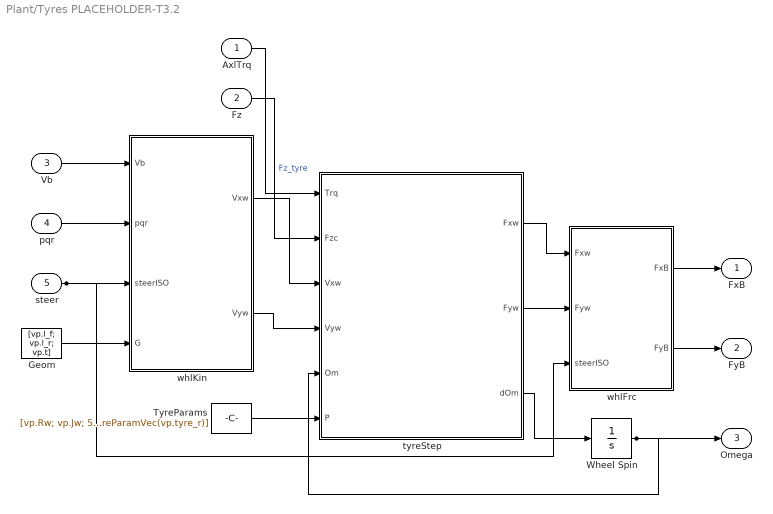
== system Plant/Tyres PLACEHOLDER-T3.2 ==
  AxlTrq : Inport
  Fz : Inport  Port=2
  Vb : Inport  Port=3
  pqr : Inport  Port=4
  steer : Inport  Port=5
  Geom : Constant  Description=Wheel-position geometry: [vp.l_f; vp.l_r; vp.t] (m).  Value=[vp.l_f; vp.l_r; vp.t]
  TyreParams : Constant  Description=|  Value=[vp.Rw; vp.Jw; 5; tyreParamVec(vp.tyre_f); tyreParamVec(vp.tyre_r)]
      | Tyre law parameters, resolved from the BASE WORKSPACE at load time so no confidential supplier coefficient is ever stored in this .slx (project confidentiality rule).
      |   1     vp.Rw   rolling radius [m]           Parameters/vehParams.m
      |   2     vp.Jw   wheel spin inertia [kg.m^2]  Parameters/vehParams.m
      |   3     VXLOW   low-speed slip guard [m/s] = 5. A NUMERICAL guard, not vehicle data.
      |           The wheel-slip mode has eigenvalue |lambda| = Cf*Rw^2/(Jw*v), i.e. it stiffens
      |           as speed falls. With the real Zenvo tyres (Cf ~ mu*Fz/s_peak ~ 6.3e4 N per unit
      |           slip at a rear corner) that is |lambda|*dt = 5.05 at v = 1 m/s and dt = 1 ms --
      |           past ode4's ~2.78 stability limit, so a launch from rest DIVERGED (measured:
      |           counter-rotating wheels, r = 82 rad/s). At 5 m/s it is 1.01, a ~2.8x margin.
      |           The VDB blocks this replaced hid the same stiffness behind their force
      |           relaxation, which this model does not carry. Inactive above 5 m/s, so it has NO
      |           effect on any lap (entry speed ~66 m/s) and none on gate 1 (which runs at 25 m/s).
      |   4-22  front axle coefficients, order defined by simulink/params/tyreParamVec.m
      |  23-41  rear  axle coefficients, same order
  Wheel Spin : Integrator  Description=|  InitialCondition=plantVx0/vp.Rw*ones(4,1)
      | Wheel spin state [FL FR RL RR], rad/s. Reproduces Scripts/vehModel.m:703-706, Jw*dOm/dt = T - fx*Rw, in the TIME domain (the offline model carries the extra sf factor only because it integrates in distance).
      | 
      | The initial condition is driven off plantVx0 -- the same model-workspace variable as the body's xbdot_o -- so a rolling start can never begin with the wheels stationary (which would put every tyre at kappa = -1 on step one).
      | 
      | This integrator also removes the direct feedthrough the VDB block had from AxlTrq to Omega. The root-level Omega Memory block is therefore no longer REQUIRED to break an algebraic loop; it is left in place because the one-step lag it applies to the inverter power cap is physically honest (see its own description) and removing it would change the solved trajectory for no gain.
  tyreStep : MATLAB Function  Description=|  TreatAsAtomicUnit=on
      | GATE-1 FALLBACK (T3.2). Direct implementation of Functions/tyreMFnum.m -- the same per-axle Pacejka MF5.2 formulas Scripts/vehModel.m's tyreMF() uses, so the plant and the offline MLTP model now share ONE tyre law by construction instead of by a coefficient conversion that provably cannot match.
      | 
      | It replaced four VDB "Combined Slip Wheel 2DOF" blocks. Gate 1 measured those reproducing tyreMFnum's Fx exactly (worst 3.8e-06) but missing Fy at 522/1592 grid points, worst 2.39e-02, ordered by distance from FNOMIN -- the PKY structural limit documented in simulink/tools/mf52ToVDB.m (MF6.2's cornering stiffness is a saturating arctangent family with no quadratic-in-Fz member, which is what tyreMFnum's load-independent By implies).
      | 
      | WHAT WAS LOST with the VDB blocks, and why it is acceptable here: tyre relaxation (first-order lag, ~5 ms at 25 m/s), the vertical/carcass model (already disabled -- vertType was None), Mx/My/Mz, turn slip, pressure and camber sensitivity. None was mapped from the MF5.2 source; all of it ran on the block's DEFAULT tyre. The offline model has none of it either, so the plant is now closer to the reference, not further.
      | 
      | CONFIDENTIALITY: no coefficient value appears in this block or anywhere in the .slx. They arrive at load time through the TyreParams constant, which holds only the expression simulink/params/tyreParamVec.m resolves.
  whlFrc : MATLAB Function  TreatAsAtomicUnit=on
  whlKin : MATLAB Function  TreatAsAtomicUnit=on
  FxB : Outport
  FyB : Outport  Port=2
  Omega : Outport  Port=3
  wires:
  Fz/1 -> tyreStep/2(Fzc)  "Fz_tyre"
  Vb/1 -> whlKin/1(Vb)
  whlKin/2(Vyw) -> tyreStep/4(Vyw)
  Geom/1 -> whlKin/4(G)
  pqr/1 -> whlKin/2(pqr)
  whlKin/1(Vxw) -> tyreStep/3(Vxw)
  steer/1 -> whlFrc/3(steerISO), whlKin/3(steerISO)
  AxlTrq/1 -> tyreStep/1(Trq)
  TyreParams/1 -> tyreStep/6(P)
  tyreStep/1(Fxw) -> whlFrc/1(Fxw)
  tyreStep/2(Fyw) -> whlFrc/2(Fyw)
  tyreStep/3(dOm) -> Wheel Spin/1
  whlFrc/1(FxB) -> FxB/1
  whlFrc/2(FyB) -> FyB/1
  Wheel Spin/1 -> tyreStep/5(Om), Omega/1

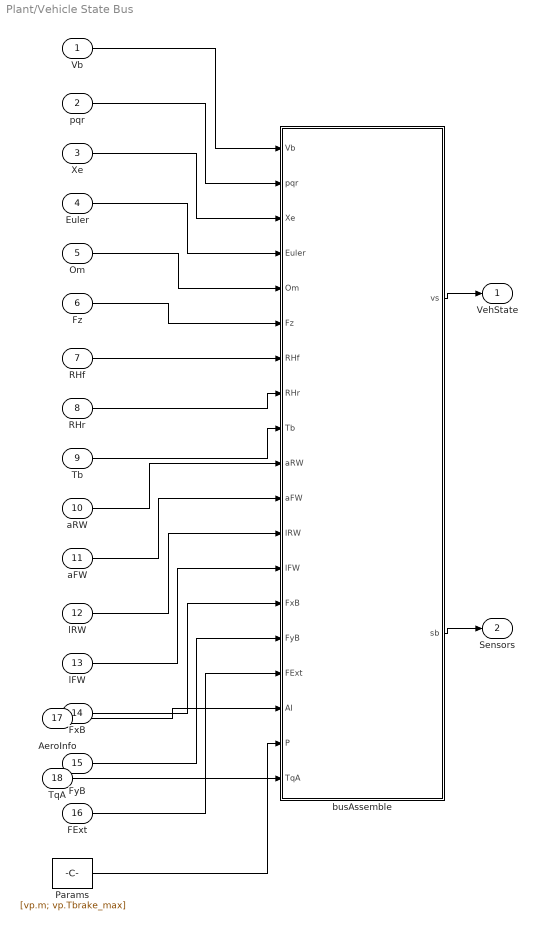
== system Plant/Vehicle State Bus ==
  Vb : Inport
  pqr : Inport  Port=2
  Xe : Inport  Port=3
  Euler : Inport  Port=4
  Om : Inport  Port=5
  Fz : Inport  Port=6
  RHf : Inport  Port=7
  RHr : Inport  Port=8
  Tb : Inport  Port=9
  aRW : Inport  Port=10
  aFW : Inport  Port=11
  lRW : Inport  Port=12
  lFW : Inport  Port=13
  FxB : Inport  Port=14
  FyB : Inport  Port=15
  FExt : Inport  Port=16
  AeroInfo : Inport  Description=Aero diagnostics 4x1 [ClF; ClR; Cd; clampCode] from the Aero subsystem (T3.4).  Port=17
  TqA : Inport  Description=Nominal pre-TV total front-axle wheel torque [Nm]. See Plant/Front Axle Trq.  Port=18
  Params : Constant  Description=|  Value=[vp.m; vp.Tbrake_max]
      | 1 vp.m           total mass [kg], for the specific-force (ax/ay) calculation
      | 2 vp.Tbrake_max  SensorBus.TbMax [Nm], POSITIVE by contract
  busAssemble : MATLAB Function  TreatAsAtomicUnit=on
  VehState : Outport
  Sensors : Outport  Port=2
  wires:
  RHf/1 -> busAssemble/7(RHf)
  Om/1 -> busAssemble/5(Om)
  Xe/1 -> busAssemble/3(Xe)
  Vb/1 -> busAssemble/1(Vb)
  RHr/1 -> busAssemble/8(RHr)
  Fz/1 -> busAssemble/6(Fz)
  Euler/1 -> busAssemble/4(Euler)
  pqr/1 -> busAssemble/2(pqr)
  Tb/1 -> busAssemble/9(Tb)
  aRW/1 -> busAssemble/10(aRW)
  aFW/1 -> busAssemble/11(aFW)
  lRW/1 -> busAssemble/12(lRW)
  lFW/1 -> busAssemble/13(lFW)
  FxB/1 -> busAssemble/14(FxB)
  FyB/1 -> busAssemble/15(FyB)
  FExt/1 -> busAssemble/16(FExt)
  busAssemble/1(vs) -> VehState/1
  busAssemble/2(sb) -> Sensors/1
  AeroInfo/1 -> busAssemble/17(AI)
  Params/1 -> busAssemble/18(P)
  TqA/1 -> busAssemble/19(TqA)

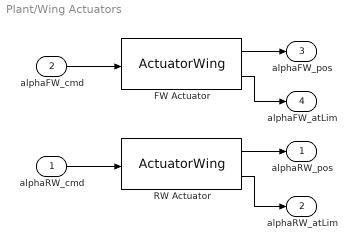
== system Plant/Wing Actuators ==
  alphaRW_cmd : Inport
  alphaFW_cmd : Inport  Port=2
  FW Actuator : AeroActuators/ActuatorWing  tau=act.tau  Ts=0.001  rateLim=act.rateLim  clamp2=act.fwClamp  alpha0=0  limTol=1e-6
  RW Actuator : AeroActuators/ActuatorWing  tau=act.tau  Ts=0.001  rateLim=act.rateLim  clamp2=act.rwClamp  alpha0=0  limTol=1e-6
  alphaRW_pos : Outport
  alphaRW_atLim : Outport  Port=2
  alphaFW_pos : Outport  Port=3
  alphaFW_atLim : Outport  Port=4
  wires:
  RW Actuator/2 -> alphaRW_atLim/1
  alphaFW_cmd/1 -> FW Actuator/1
  alphaRW_cmd/1 -> RW Actuator/1
  FW Actuator/2 -> alphaFW_atLim/1
  FW Actuator/1 -> alphaFW_pos/1
  RW Actuator/1 -> alphaRW_pos/1

== matlab function Plant/Vehicle State Bus/busAssemble ==
  data: Vb input; vs output Bus: VehStateBus; pqr input; Xe input; Euler input; Om input; Fz input; RHf input; RHr input; Tb input; aRW input; aFW input; lRW input; lFW input; FxB input; FyB input; FExt input; AI input; P input; sb output Bus: SensorBus; TqA input
function [vs, sb] = busAssemble(Vb, pqr, Xe, Euler, Om, Fz, RHf, RHr, Tb, ...
                                aRW, aFW, lRW, lFW, FxB, FyB, FExt, AI, P, TqA)
%#codegen
% Assemble VehStateBus (vs) and SensorBus (sb), applying the SAE -> ISO 8855
% mirror. This is the ONLY place the flip happens.
%
%   y, vy, ay, psi, r, z, roll  all NEGATE     (y RIGHT -> y LEFT, z DOWN -> z UP)
%   x, vx, ax, pitch            unchanged      (the mirror is about the x-z plane)
%   corner labels fl/fr/rl/rr   unchanged      (physical, not a vector component)
%
% ax/ay are SPECIFIC FORCE (what an accelerometer at the CG reads, gravity
% excluded): the sum of the tyre body-frame forces plus the aero external force,
% over the mass. Exact -- no differentiation of a state.
%
% AI = the Aero subsystem's 4x1 diagnostics [ClF; ClR; Cd; clampCode] (T3.4).
% They are FRAME-FREE scalars (coefficients and a bit code), so the SAE -> ISO
% mirror does not touch them.
%
% P = [m; Tbrake_max]

mm = P(1); Tbmax = P(2);

sumFx = FxB(1) + FxB(2) + FxB(3) + FxB(4) + FExt(1);
sumFy = FyB(1) + FyB(2) + FyB(3) + FyB(4) + FExt(2);

vs.vx    =  Vb(1);
vs.vy    = -Vb(2);
vs.r     = -pqr(3);
vs.ax    =  sumFx/mm;
vs.ay    = -sumFy/mm;
vs.x     =  Xe(1);
vs.y     = -Xe(2);
vs.psi   = -Euler(3);
vs.z     = -Xe(3);
vs.roll  = -Euler(1);
vs.pitch =  Euler(2);
vs.RHf   =  RHf;
vs.RHr   =  RHr;
vs.Om_fl =  Om(1);
vs.Om_fr =  Om(2);
vs.Om_rl =  Om(3);
vs.Om_rr =  Om(4);
vs.Fz_fl =  Fz(1);
vs.Fz_fr =  Fz(2);
vs.Fz_rl =  Fz(3);
vs.Fz_rr =  Fz(4);
vs.Tbrake_applied = Tb;
vs.alphaRW_pos    = aRW;
vs.alphaFW_pos    = aFW;
% the ActuatorWing library block emits at_limit as LOGICAL; VehStateBus carries
% it as double, so cast once here rather than changing the bus or the library.
vs.alphaRW_atLim  = double(lRW);
vs.alphaFW_atLim  = double(lFW);
vs.aeroClF        = AI(1);
vs.aeroClR        = AI(2);
vs.aeroCd         = AI(3);
vs.aeroClamp      = AI(4);
% Per-corner LATERAL tyre force (T4.2, review fix I2). FyB is the body-frame
% SAE (y RIGHT) lateral force per corner, so it takes the same negation as
% vy/ay/y above -- this is still the only place the SAE->ISO flip happens.
% Published because a consumer that needs per-axle lateral force otherwise has
% to assume the STATIC l_r/l : l_f/l split of m*ay, which is wrong precisely
% where it is used: lateral load transfer and the front/rear aero balance both
% move the real split, and the aero balance is a controlled variable here.
% FExt(2) (the aero side force) is deliberately NOT distributed into these --
% they are TYRE forces, and vs.ay above remains the whole-vehicle quantity.
vs.Fy_fl = -FyB(1);
vs.Fy_fr = -FyB(2);
vs.Fy_rl = -FyB(3);
vs.Fy_rr = -FyB(4);

% SensorBus contract (Functions/rwVelocityTarget.m brakeSwitch): Tbrake SIGNED
% (<= 0 braking, the law applies tbSign = -1 itself and avoids abs() on purpose),
% TbMax the POSITIVE magnitude cap. TbMax > 0 ALWAYS -- the onset width is
% w1frac*TbMax.
sb.vx     =  Vb(1);
sb.r      = -pqr(3);
sb.Tbrake =  Tb;
sb.TbMax  =  Tbmax;
% kappaRef (T4.2): the PLANT HAS NO PATH KNOWLEDGE, so it publishes 0 here and
% the harness substitutes the driver value -- ARFWr_Sim/ECU Sensor Latency takes
% vx/r/Tbrake/TbMax/TqAxle off this bus but sources element 5 from DriverPath's
% preview-curvature outport. It is NOT omitted from the struct: Plant's Sensors
% outport is typed Bus: SensorBus and every element must be assigned.
% Standalone Plant runs (and ARFWr_Replay) therefore see kappaRef = 0, which makes
% the TV allocator a no-op -- its error is kappaRef*vx - r, and with no path
% reference the only defensible target is zero commanded yaw rate.
sb.kappaRef = 0;
% TqAxle (T4.2): nominal PRE-TV total front-axle wheel torque [Nm], drive + brake,
% signed. See Plant/Front Axle Trq for why AxlTrq(1)+AxlTrq(2) is exactly the
% pre-TV quantity tvAllocStep.m's headroom clamp expects.
sb.TqAxle   = TqA;

== matlab function Plant/Tyres PLACEHOLDER-T3.2/tyreStep ==
  data: Trq input; Fxw output; Fzc input; Vxw input; Vyw input; Om input; P input; Fyw output; dOm output
function [Fxw, Fyw, dOm] = tyreStep(Trq, Fzc, Vxw, Vyw, Om, P)
%#codegen
% Per-corner Pacejka MF5.2 tyre forces + wheel-spin derivative.
%
% GATE-1 FALLBACK (T3.2). The formulas below are Functions/tyreMFnum.m
% transcribed verbatim -- the numeric twin of Scripts/vehModel.m's tyreMF().
% KEEP ALL THREE IDENTICAL. This is the same twin-formula rule the repo
% already applies to aeroEvalSX/aeroEvalNum and tyreMF/tyreMFnum.
%
% Corner order is [FL; FR; RL; RR]; corners 1-2 use the FRONT coefficient
% block, 3-4 the REAR one -- one parameter set per axle, which is the
% granularity of the supplier data (vp.tyre_f / vp.tyre_r).
%
% FRAME. Vxw/Vyw are contact-patch velocities already rotated into each
% WHEEL frame by whlKin, and Fxw/Fyw are returned in that same wheel frame
% for whlFrc to rotate back. The sign relationship reproduced here is the
% one MEASURED on the VDB block it replaces: with slip angle taken as
% alpha = atan(Vyw/Vxw), the block's Fy has the SAME sign as tyreMFnum's fy
% at that alpha (measured ratio +0.871 at alpha = +5 deg before the fallback,
% i.e. same sign, magnitude short by the PKY structural error). Nothing
% outside this block therefore changes sign, and the lap that T2.3 already
% drove stays valid.
%
% P = [Rw; Jw; VXLOW; front(19); rear(19)], order owned by
% simulink/params/tyreParamVec.m.

Rw    = P(1);
Jw    = P(2);
VXLOW = P(3);

Fxw = zeros(4,1);
Fyw = zeros(4,1);
dOm = zeros(4,1);

for i = 1:4
    if i <= 2
        o = 3;          % front coefficients start at P(4)
    else
        o = 3 + 19;     % rear coefficients start at P(23)
    end

    Fz0  = P(o+1);
    pDx1 = P(o+2);  pDx2 = P(o+3);
    Bx   = P(o+4);  Cx   = P(o+5);  Ex = P(o+6);
    pDy1 = P(o+7);  pDy2 = P(o+8);
    By   = P(o+9);  Cy   = P(o+10); Ey = P(o+11);
    rBx1 = P(o+12); rBx2 = P(o+13); rCx1 = P(o+14); rEx1 = P(o+15);
    rBy1 = P(o+16); rBy2 = P(o+17); rCy1 = P(o+18); rEy1 = P(o+19);

    % Low-speed guard. The offline model divides by the contact-patch
    % longitudinal speed outright (vehModel.m:634) because its NLP never
    % visits standstill; a plant that starts from rest must. VXLOW is the
    % same 1 m/s floor the VDB block used for its own regularisation, and it
    % is inactive above that speed, so it changes nothing the gate measured.
    vx = Vxw(i);
    vs = abs(vx);
    if vs < VXLOW
        vs = VXLOW;
    end

    sx = (Rw*Om(i) - vx) / vs;

    % SLIP-ANGLE SIGN. Scripts/vehModel.m works in ISO 8855 (y LEFT) and forms
    % the rear slip angle as sa = atan((l_r*r - vy)/vx) = -atan(vy_corner/vx),
    % i.e. the NEGATIVE of the corner's lateral-velocity angle, so that a
    % wheel sliding left generates force to the right. This subsystem works in
    % SAE (y RIGHT), which mirrors vy but NOT the required opposition, so the
    % same minus sign must appear here. Without it the lateral force acts along
    % the slip velocity instead of against it: the yaw moment at zero steer
    % becomes +l_f*f(r*l_f) + l_r*f(r*l_r), which is POSITIVE FEEDBACK.
    % Measured with the sign omitted: a zero-steer launch diverged to
    % r = 80 rad/s with counter-rotating wheels. An exactly symmetric run
    % (rolling start, no steer) does NOT reveal it -- vy and r stay identically
    % zero, so there is nothing for the wrong sign to amplify.
    % Gxa and Gyk are EVEN in sa, so this sign affects fy0 only, exactly as
    % it does in Functions/tyreMFnum.m.
    sa = -atan(Vyw(i) / vs);

    fz  = Fzc(i);
    if fz < 0
        fz = 0;          % a lifted wheel carries no load and makes no force
    end

    dfz = (fz - Fz0) / Fz0;
    mux = pDx1 + pDx2*dfz;
    muy = pDy1 + pDy2*dfz;

    % pure slip
    fx0 = mux*fz*sin(Cx*atan(Bx*sx - Ex*(Bx*sx - atan(Bx*sx))));
    fy0 = muy*fz*sin(Cy*atan(By*sa - Ey*(By*sa - atan(By*sa))));

    % combined-slip weighting
    Bxa = rBx1*cos(atan(rBx2*sx));
    Gxa = cos(rCx1*atan(Bxa*sa - rEx1*(Bxa*sa - atan(Bxa*sa))));
    Byk = rBy1*cos(atan(rBy2*sa));
    Gyk = cos(rCy1*atan(Byk*sx - rEy1*(Byk*sx - atan(Byk*sx))));

    % VALIDITY GUARD -- required by a plant that starts from rest; inactive
    % anywhere the offline model operates, so the two stay identical there.
    % Gxa/Gyk are Pacejka combined-slip WEIGHTING factors: physically they
    % lie in [0,1] and only ever REDUCE the pure-slip force. Their cosine
    % form only respects that for moderate slip -- once |sx| grows past a few
    % tenths the atan argument saturates and cos() can go NEGATIVE, which
    % REVERSES the force instead of shrinking it. The NLP never visits that
    % region (its slips stay small), but a plant accelerating from standstill
    % does: with vx below the VXLOW floor, sx = Rw*Om - vx reaches O(1-100)
    % within the first few steps of wheelspin. Measured without this clamp:
    % Gyk flipped sign, the left and right tyres pulled opposite ways, and a
    % zero-steer 25%-throttle run from rest diverged to r = 82 rad/s with the
    % wheels counter-rotating. Clamping to [0,1] makes a spinning tyre simply
    % lose its lateral force, which is the correct physical limit.
    Gxa = min(max(Gxa, 0), 1);
    Gyk = min(max(Gyk, 0), 1);

    Fxw(i) = Gxa*fx0;
    Fyw(i) = Gyk*fy0;

    % wheel spin, vehModel.m:703-706 without the distance-domain sf factor
    dOm(i) = (Trq(i) - Fxw(i)*Rw) / Jw;
end
